simulink model "minor_project"  (R2018a)
settings: Solver=VariableStepAuto  StartTime=0.0  StopTime=0.2  RelTol=1e-3
libraries: powerlib x8, dspstat3 x1
settings Model: Creator=DaniShah  LastModifiedBy=DaniShah

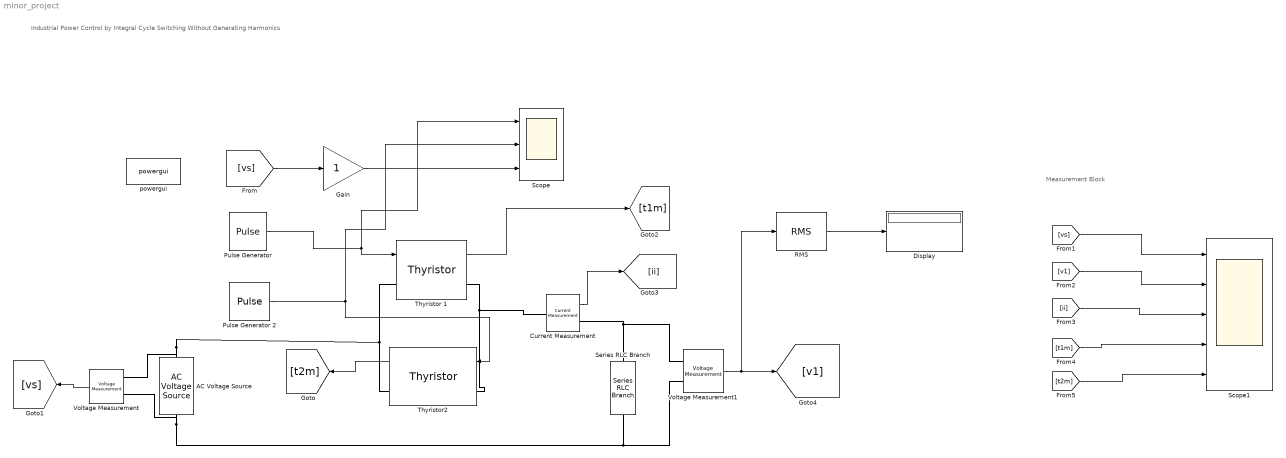
== system minor_project ==
  note: Measurement Block
  note: Industrial Power Control by Integral Cycle Switching Without Generating Harmonics
  AC Voltage Source : powerlib/Electrical Sources/AC Voltage Source  Amplitude=230  Phase=0  Frequency=50  SampleTime=0  Measurements=None  BusType=swing  Pref=10e3  Qref=0  Qmin=-inf  Qmax=+inf
  Current Measurement : powerlib/Measurements/Current Measurement  PhasorSimulation=off  OutputType=Complex  PSBequivalent=0
  Display : Display
  Gain : Gain
  Pulse Generator : DiscretePulseGenerator  PulseType=Time based  Amplitude=10  Period=0.1  PulseWidth=6  PhaseDelay=0.005
  Pulse Generator 2 : DiscretePulseGenerator  PulseType=Time based  Amplitude=10  Period=0.1  PulseWidth=6  PhaseDelay=0.005
  RMS : dspstat3/RMS  run=off  directionMode=Each column  dimension=1  InputProcessing=Columns as channels (frame based)  reset_popup=None
  Scope : Scope  NumInputPorts=3
  Scope1 : Scope  NumInputPorts=5
  Series RLC Branch : powerlib/Elements/Series RLC Branch  LConnTagsString=__new0  RConnTagsString=__new0  BranchType=R  Resistance=100  Inductance=1e-3  SetiL0=off  InitialCurrent=0  Capacitance=1e-6  Setx0=off  InitialVoltage=0  Measurements=None
  Thyristor 1 : powerlib/Power Electronics/Thyristor  Ron=1  Lon=0  Vf=0.8  IC=0  Rs=500  Cs=250e-9  Measurements=on
  Thyristor2 : powerlib/Power Electronics/Thyristor  Ron=1  Lon=0  Vf=0.8  IC=0  Rs=500  Cs=250e-9  Measurements=on
  Voltage Measurement : powerlib/Measurements/Voltage Measurement  PhasorSimulation=off  OutputType=Complex  PSBequivalent=0
  Voltage Measurement1 : powerlib/Measurements/Voltage Measurement  PhasorSimulation=off  OutputType=Complex  PSBequivalent=0
  powergui : powerlib/powergui  Priority=1  SimulationMode=Continuous  SampleTime=50e-6  frequency=60  Iterations=50  frequencyindice=50  Pbase=100e6  ErrMax=1e-4  UnitsV=kV  UnitsW=MW  buscounter=0  FunctionMessages=off  echomessages=off  EnableUseOfTLC=off  CurrentSourceSwitches=off  DisableSnubberDevices=off  DisableRonSwitches=off  DisableVfSwitches=off  DisplayEquations=off  SolverType=Tustin/Backward Euler (TBE)  Interpol=off  ExternalGateDelay=off  methode=off  Ts=100  x0status=blocks  SPID=on  SwTol=0  HookPort=off  RestoreLinks=warning  ResistiveCurrentMeasurement=off  Frange=[0:2:500]  Ylog=off  Xlog=on  ShowGrid=off  save=off  variable=ZData  structure=0  ZoomFFT=off  StartTime=0.0  cycles=1  DisplayStyle=1  fundamental=60  FreqAxis=off  MaxFrequency=1000  frequencyindicesteady=1  RmsSteady=1  display=off
  wires:
  [vs] -> Gain/1
  Gain/1 -> Scope/3
  Pulse Generator/1 -> Scope/1, Thyristor 1/1
  Pulse Generator 2/1 -> Thyristor2/1, Scope/2
  Thyristor2/1 -> [t2m]
  Voltage Measurement/1 -> [vs]
  Thyristor 1/1 -> [t1m]
  Current Measurement/1 -> [ii]
  Voltage Measurement1/1 -> RMS/1, [v1]
  RMS/1 -> Display/1
  [vs] -> Scope1/1
  [v1] -> Scope1/2
  [ii] -> Scope1/3
  [t1m] -> Scope1/4
  [t2m] -> Scope1/5
  connections:
  Thyristor2/RConn1 -- Voltage Measurement/LConn1 -- AC Voltage Source/RConn1 -- Thyristor 1/LConn1
  Thyristor 1/RConn1 -- Current Measurement/LConn1 -- Thyristor2/LConn1
  Voltage Measurement/LConn2 -- Series RLC Branch/RConn1 -- Voltage Measurement1/LConn2 -- AC Voltage Source/LConn1
  Voltage Measurement1/LConn1 -- Series RLC Branch/LConn1 -- Current Measurement/RConn1
